simulink model "Nimbus_Sizing_1DOF"  (R2022a)
settings: Solver=VariableStepAuto  StartTime=0.0  StopTime=50  MaxStep=0.001  RelTol=1e-3
values from neighbouring files (symbols this model uses):
  A = (pi*D^2)/4    (= 0.0283528736986)    [Nimbus_Sizing_1DOF_var.m]
  A_drogue = (pi*D_drogue^2)/4    (= 1.1689866264)    [Nimbus_Sizing_1DOF_var.m]
  A_e = pi*(D_e/2000)^2    (= 0.00282743338823)    [Nimbus_Sizing_1DOF_var.m]
  A_para = (pi*D_para^2)/4    (= 29.22466566)    [Nimbus_Sizing_1DOF_var.m]
  Cd = 0.80    (= 0.8)    [Nimbus_Sizing_1DOF_var.m]
  Cd_para = 0.97    [Nimbus_Sizing_1DOF_var.m]
  g = 9.81    [Nimbus_Sizing_1DOF_var.m]
  m0_fuel = m0_ox/OF    (= 2.33333333333)    [Nimbus_Sizing_1DOF_var.m]
  m0_ox = 7    [Nimbus_Sizing_1DOF_var.m]
  m_f_dot = (T/V_e)*(1/(OF+1))    (= 0.347511815402)    [Nimbus_Sizing_1DOF_var.m]
  m_ox_dot = (T/V_e)*(OF/(OF+1))    (= 1.04253544621)    [Nimbus_Sizing_1DOF_var.m]
  p0 = 101325    [Nimbus_Sizing_1DOF_var.m]
  R = 287    [Nimbus_Sizing_1DOF_var.m]
  V_e = g*Isp    (= 2158.2)    [Nimbus_Sizing_1DOF_var.m]
settings Model: SimulationMode=accelerator  Creator=marti  LastModifiedBy=usmaanyaqoob
settings SolverCC: MaxConsecutiveMinStep=5
settings DebuggingCC: UnconnectedInputMsg=warning  UnconnectedOutputMsg=warning  UnconnectedLineMsg=warning  SFMachineParentedDataDiag=warning
settings RTWCC: DLArmComputeVersion=19.05

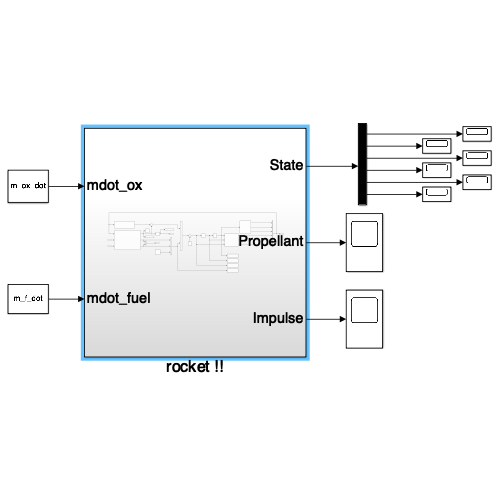
[thumbnail: Simulink's stored preview of the top-level diagram]
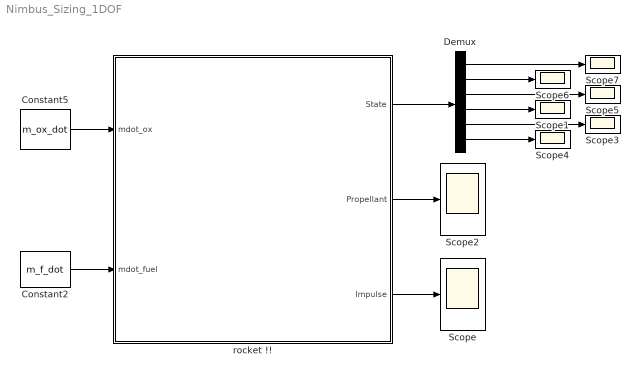
== system Nimbus_Sizing_1DOF ==
  Constant2 : Constant  Value=m_f_dot
  Constant5 : Constant  Value=m_ox_dot
  Demux : Demux  Outputs=6
  Scope{,1..7} (8 alike) : Scope
  rocket !! : Subsystem
  wires:
  rocket !!/3(Impulse) -> Scope/1
  Constant2/1 -> rocket !!/2(mdot_fuel)
  Constant5/1 -> rocket !!/1(mdot_ox)
  rocket !!/2(Propellant) -> Scope2/1
  rocket !!/1(State) -> Demux/1
  Demux/4 -> Scope1/1
  Demux/5 -> Scope3/1
  Demux/6 -> Scope4/1
  Demux/3 -> Scope5/1
  Demux/2 -> Scope6/1
  Demux/1 -> Scope7/1

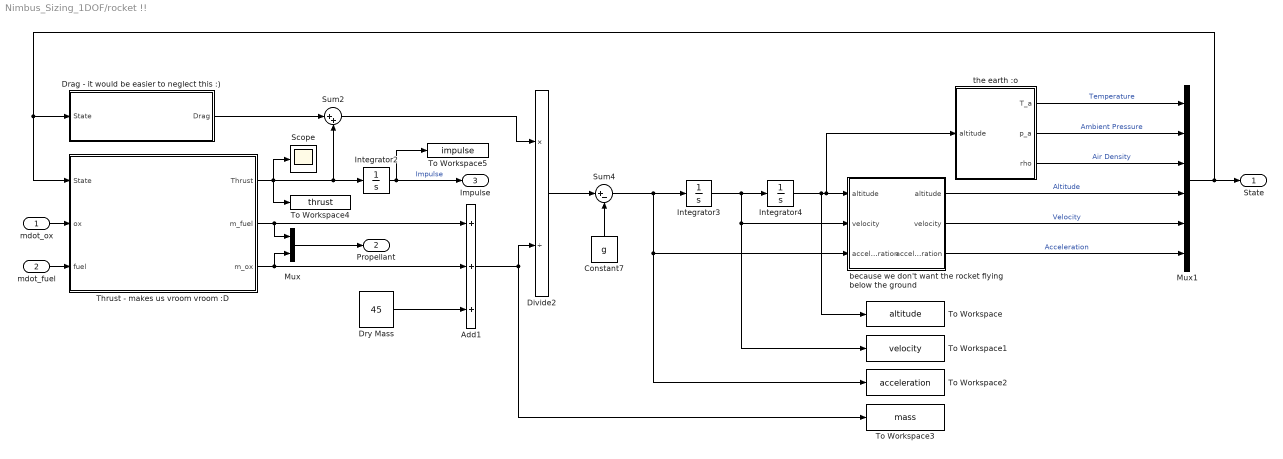
== system Nimbus_Sizing_1DOF/rocket !! ==
  mdot_ox : Inport
  mdot_fuel : Inport  Port=2
  "  the earth :o" : MATLAB Function  TreatAsAtomicUnit=on
  Add1 : Sum  Inputs=+++
  Constant7 : Constant  Value=g
  Divide2 : Product  Inputs=*/
  "Drag - it would be easier to neglect this :) " : Subsystem
  Dry Mass : Constant  Value=45
  Integrator2 : Integrator
  Integrator3 : Integrator
  Integrator4 : Integrator
  Mux : Mux  Inputs=2
  Mux1 : Mux  Inputs=6
  Scope : Scope
  Sum2 : Sum  Inputs=|++
  Sum4 : Sum  Inputs=|+-
  Thrust - makes us vroom vroom :D : Subsystem
  To Workspace : ToWorkspace  VariableName=altitude  SaveFormat=Timeseries  SampleTime=-1
  To Workspace1 : ToWorkspace  VariableName=velocity  SaveFormat=Timeseries  SampleTime=-1
  To Workspace2 : ToWorkspace  VariableName=acceleration  SaveFormat=Timeseries  SampleTime=-1
  To Workspace3 : ToWorkspace  VariableName=mass  SaveFormat=Timeseries  SampleTime=-1
  To Workspace4 : ToWorkspace  VariableName=thrust  SaveFormat=Timeseries  SampleTime=-1
  To Workspace5 : ToWorkspace  VariableName=impulse  SaveFormat=Timeseries  SampleTime=-1
  because we don't want the rocket flying below the ground : MATLAB Function  TreatAsAtomicUnit=on
  State : Outport
  Propellant : Outport  Port=2
  Impulse : Outport  Port=3
  wires:
  Dry Mass/1 -> Add1/3
  Thrust - makes us vroom vroom :D/3(m_ox) -> Add1/2, Mux/2
  Thrust - makes us vroom vroom :D/2(m_fuel) -> Add1/1, Mux/1
  Add1/1 -> To Workspace3/1, Divide2/2
  mdot_fuel/1 -> Thrust - makes us vroom vroom :D/3(fuel)
  mdot_ox/1 -> Thrust - makes us vroom vroom :D/2(ox)
  "Drag - it would be easier to neglect this :) "/1(Drag) -> Sum2/1
  Sum2/1 -> Divide2/1
  Divide2/1 -> Sum4/1
  Constant7/1 -> Sum4/2
  Sum4/1 -> because we don't want the rocket flying below the ground/3("acceleration "), To Workspace2/1, Integrator3/1
  Integrator3/1 -> To Workspace1/1, because we don't want the rocket flying below the ground/2("velocity "), Integrator4/1
  Mux1/1 -> State/1, Thrust - makes us vroom vroom :D/1(State), "Drag - it would be easier to neglect this :) "/1(State)
  Thrust - makes us vroom vroom :D/1(Thrust) -> To Workspace4/1, Scope/1, Integrator2/1, Sum2/2
  Integrator2/1 -> To Workspace5/1, Impulse/1  "Impulse"
  "  the earth :o"/1(T_a) -> Mux1/1  "Temperature"
  "  the earth :o"/2(p_a) -> Mux1/2  "Ambient Pressure"
  "  the earth :o"/3(rho) -> Mux1/3  "Air Density"
  Mux/1 -> Propellant/1
  because we don't want the rocket flying below the ground/1(altitude) -> Mux1/4  "Altitude"
  Integrator4/1 -> "  the earth :o"/1(altitude), because we don't want the rocket flying below the ground/1("altitude "), To Workspace/1
  because we don't want the rocket flying below the ground/2(velocity) -> Mux1/5  "Velocity"
  because we don't want the rocket flying below the ground/3(acceleration) -> Mux1/6  "Acceleration"

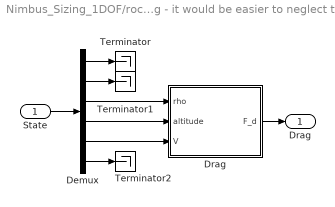
== system Nimbus_Sizing_1DOF/rocket !!/Drag - it would be easier to neglect this :)  ==
  State : Inport
  Demux : Demux  Outputs=6
  "Drag " : MATLAB Function  TreatAsAtomicUnit=on
  Terminator : Terminator
  Terminator1 : Terminator
  Terminator2 : Terminator
  Drag : Outport
  wires:
  "Drag "/1(F_d) -> Drag/1
  State/1 -> Demux/1
  Demux/1 -> Terminator/1
  Demux/2 -> Terminator1/1
  Demux/6 -> Terminator2/1
  Demux/3 -> "Drag "/1(rho)
  Demux/4 -> "Drag "/2(altitude)
  Demux/5 -> "Drag "/3(V)

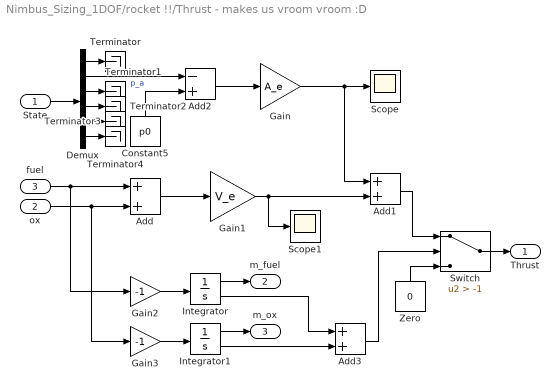
== system Nimbus_Sizing_1DOF/rocket !!/Thrust - makes us vroom vroom :D ==
  State : Inport
  ox : Inport  Port=2
  fuel : Inport  Port=3
  Add : Sum
  Add1 : Sum
  Add2 : Sum  Inputs=-+
  Add3 : Sum
  Constant5 : Constant  Value=p0
  Demux : Demux  Outputs=6
  Gain : Gain  Gain=A_e
  Gain1 : Gain  Gain=V_e
  Gain2 : Gain  Gain=-1
  Gain3 : Gain  Gain=-1
  Integrator : Integrator  InitialCondition=m0_fuel  LimitOutput=on  LowerSaturationLimit=0  ShowSaturationPort=on
  Integrator1 : Integrator  InitialCondition=m0_ox  LimitOutput=on  LowerSaturationLimit=0  ShowSaturationPort=on
  Scope : Scope
  Scope1 : Scope
  Switch : Switch  Criteria=u2 > Threshold  Threshold=-1  SaturateOnIntegerOverflow=off  InputSameDT=off
  Terminator{,1..4} (5 alike) : Terminator
  Zero : Constant  Value=0  OutDataTypeStr=Inherit: Inherit via back propagation
  Thrust : Outport
  m_fuel : Outport  Port=2
  m_ox : Outport  Port=3
  wires:
  fuel/1 -> Add/1, Gain2/1
  ox/1 -> Gain3/1, Add/2
  Add2/1 -> Gain/1
  Add/1 -> Gain1/1
  Constant5/1 -> Add2/2
  Demux/2 -> Add2/1  "p_a"
  Gain1/1 -> Scope1/1, Add1/2
  Gain/1 -> Add1/1, Scope/1
  Add1/1 -> Switch/1
  Integrator/1 -> m_fuel/1
  Gain2/1 -> Integrator/1
  Integrator1/1 -> m_ox/1
  Gain3/1 -> Integrator1/1
  State/1 -> Demux/1
  Demux/3 -> Terminator1/1
  Demux/1 -> Terminator/1
  Demux/4 -> Terminator2/1
  Demux/6 -> Terminator4/1
  Demux/5 -> Terminator3/1
  Zero/1 -> Switch/3
  Switch/1 -> Thrust/1
  Integrator/2 -> Add3/1
  Integrator1/2 -> Add3/2
  Add3/1 -> Switch/2

== matlab function Nimbus_Sizing_1DOF/rocket !!/because we don't want the rocket flying below the ground ==
  data: altitude input; altitude output; velocity input; acceleration input; velocity output; acceleration output
function [altitude,velocity,acceleration] = fcn(altitude,velocity,acceleration)

if altitude <= 0
    altitude = 0;
    velocity = 0;
    acceleration = 0;
end

== matlab function Nimbus_Sizing_1DOF/rocket !!/Drag - it would be easier to neglect this :) /Drag  ==
  data: rho input; altitude input; V input; F_d output; Cd parameter; A parameter; Cd_para parameter; A_para parameter; A_drogue parameter
function F_d = fcn(rho, altitude, V, Cd, A, Cd_para, A_para, A_drogue)
if V > -15
    F_d = 0.5*A*rho*Cd*V^2; % Calculate drag for ascent
else
    if altitude > 1500
        F_d = 0.5*A*rho*Cd*V^2 + 0.5*A_drogue*rho*Cd_para*V^2; % Calculate drag for rocket + drogue parachute
    else
        F_d = 0.5*A*rho*Cd*V^2 + 0.5*A_para*rho*Cd_para*V^2; % Calculate drag for rocket + main parachute
    end
end

% Direction correction based on sign of velocity
if V > 0
    F_d = F_d * -1;
end

== matlab function Nimbus_Sizing_1DOF/rocket !!/  the earth :o ==
  data: altitude input; T_a output; p_a output; rho output; p0 parameter; R parameter; g parameter
function [T_a, p_a, rho] = atmosphere(altitude, p0, R, g)

T0 = 288.15;
L0 = -0.0065; 

T_a = T0 + L0*altitude;
p_a = p0*(T_a/T0)^(-g/(R*L0));

rho = p_a/(0.2869*T_a*1000);
